simulink model "GFM_29bus"  (R2019a)
settings: Solver=ode1  StartTime=0.0  StopTime=4.5  FixedStep=Time_Step  RelTol=1e-3  EnableMultiTasking=on
PreLoadFcn:
  | Init_29bus;
InitFcn:
  | Init_29bus;
undefined symbols (not defined in the file): D1, D11, Delta, Time_Step, VSC01_Delta_P_Time_Step, VSC01_Delta_P_Value
libraries: powerlib x175, GFM_Lib x1
(part 1 of 5)
Description:
  | Copyright 2008-2017 The MathWorks, Inc.
settings Model: Creator=MathWorks  LastModifiedBy=Frederic_Colas
settings DataIOCC: SaveFormat=StructureWithTime  SignalLoggingSaveFormat=ModelDataLogs  SaveOutput=off  SignalLogging=off  DSMLogging=off  SaveTime=off  ReturnWorkspaceOutputs=off
settings OptimizationCC: ExpressionDepthLimit=2147483647  LifeSpan=inf
settings DebuggingCC: UnderspecifiedInitializationDetection=Classic  MergeDetectMultiDrivingBlocksExec=none  SolverPrmCheckMsg=warning  FcnCallInpInsideContextMsg=warning  UnconnectedInputMsg=none  UnconnectedOutputMsg=none  UnconnectedLineMsg=none  StateNameClashWarn=warning  SFUnexpectedBacktrackingDiag=warning  SFNoUnconditionalDefaultTransitionDiag=warning  SFExecutionAtInitializationDiag=none  ArithmeticOperatorsInVariantConditions=warning
settings HardwareCC: ProdBitPerPointer=32  ProdBitPerSizeT=32  ProdBitPerPtrDiffT=32  ProdLargestAtomicFloat=None  ProdIntDivRoundTo=Undefined  ProdEndianess=Unspecified  ProdWordSize=32  ProdHWDeviceType=32-bit Generic
settings ModelReferenceCC: PropagateSignalLabelsOutOfModel=off
settings SFSimCC: SimUseLocalCustomCode=off
settings RTWCC: RTWUseLocalCustomCode=off
settings CodeAppCC: StateflowObjectComments=on
settings GRTTargetCC: TargetLangStandard=C89/C90 (ANSI)  CombineOutputUpdateFcns=off  GRTInterface=on
settings ConfigComp: CovMetricSettings=dw  CovSaveCumulativeToWorkspaceVar=on  CovSaveSingleToWorkspaceVar=on  CovExternalEMLEnable=off  CovSFcnEnable=off
settings SimscapeCC: SimscapeNormalizeSystem=off

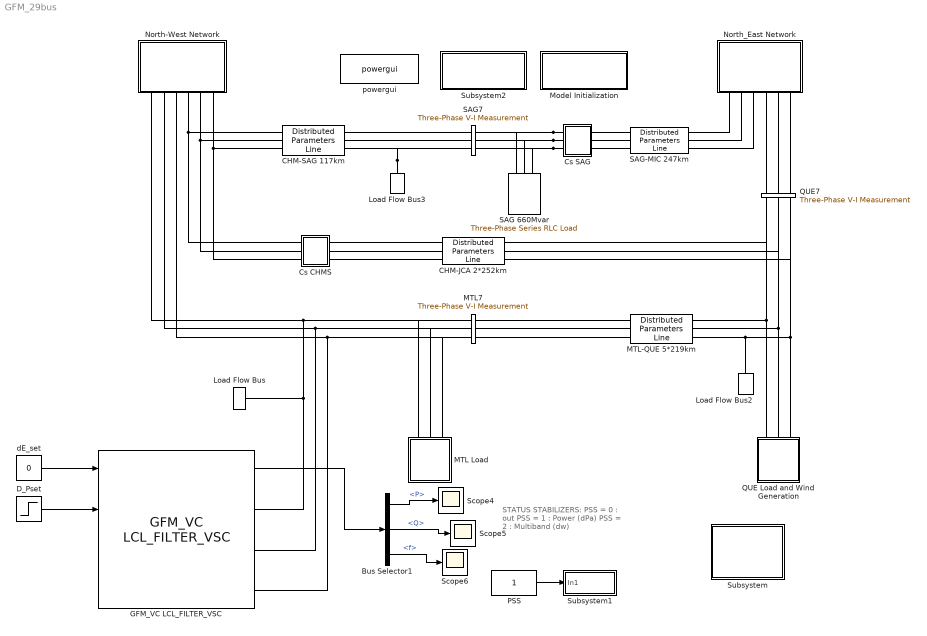
== system GFM_29bus ==
  note: STATUS STABILIZERS:
      | PSS = 0 :  out
      | PSS = 1 :  Power (dPa)
      | PSS = 2 :  Multiband (dw)
  Bus Selector1 : BusSelector  OutputSignals=P,Q,f
  CHM-JCA 2*252km : powerlib/Elements/Distributed Parameters Line  Phases=3  Length=252  Frequency=60  Resistance="[0.01273  0.3864]/2"  Inductance="[0.9337e-3  4.1264e-3]/2"  Capacitance=[12.74e-9 7.751e-9]*2  x1=[-0.00144 -2.67597627648881e-08 0 0;-0.0014 -2.6378453251211e-08 0 0;-0.00136 -2.59911455047426e-08 0 0;-0.00132 -2.55979275959245e-08 0 0;-0.00128 -2.51988889391182e-08 0 0;-0.00124 -2.47941202722731e-08 0 0;-0.0012 -2.43837136362936e-08 0 0;-0.00116 -2.39677623541093e-08 0 0;-0.00112 -2.35463610094548e-08 0 0;-0.00108 -2.3119605425362e-08 0 0;-0.00104 -2.26875926423704e-08 0 0;-0.001 -2.22504208964615e-08 0 0;-0.00096 -2.18081895967201e-08 0 0;-0.00092 -2.13609993027303e-08 0 0;-0.00088 -2.09089517017084e-08 236942.352172574 -735004.326361009;-0.00084 -2.04521495853807e-08 247998.624561456 -731347.868692905;-0.0008 -1.99906968266091e-08 258998.504201761 -727525.108826337;-0.00076 -1.95246983557715e-08 269939.48981572 -723536.916023931;-0.00072 -1.90542601369017e-08 280819.093517553 -719384.197166337;-0.00068 -1.85794891435937e-08 291634.841379201 -715067.896546013;-0.00064 -1.81004933346771e-08 302384.273992871 -710588.995652497;-0.0006 -1.76173816296682e-08 313064.947030286 -705948.512949229;-0.00056 -1.71302638840026e-08 323674.431798503 -701147.503641956;-0.00052 -1.66392508640548e-08 334210.315792179 -696187.059438794;-0.00048 -1.61444542219513e-08 344670.203242151 -691068.308301977;-0.00044 -1.56459864701817e-08 355051.715660215 -685792.414191371;-0.0004 -1.51439609560139e-08 365352.492379973 -680360.576799801;-0.00036 -1.46384918357207e-08 375570.19109363 -674774.031280245;-0.00032 -1.4129694048621e-08 385702.488384611 -669034.04796498;-0.00028 -1.3617683290944e-08 395747.080255891 -663141.932076712;-0.00024 -1.31025759895205e-08 405701.682653897 -657099.023431781;-0.0002 -1.25844892753088e-08 415564.031987891 -650906.696135503;-0.00016 -1.20635409567599e-08 425331.885644682 -644566.358269704;-0.00012 -1.1539849493029e-08 435003.022498583 -638079.451572539;-8e-05 -1.10135339670388e-08 444575.243416475 -631447.451110648;-4e-05 -1.04847140584011e-08 454046.371757867 -624671.864943746]  x2=[-0.00144 -1.4600860870236e-08 0 0;-0.0014 -1.43294294717049e-08 0 0;-0.00136 -1.40547396844836e-08 0 0;-0.00132 -1.37768539706611e-08 0 0;-0.00128 -1.34958355190521e-08 0 0;-0.00124 -1.32117482308293e-08 0 0;-0.0012 -1.2924656704992e-08 0 0;-0.00116 -1.26346262236775e-08 0 0;-0.00112 -1.23417227373161e-08 0 0;-0.00108 -1.20460128496347e-08 0 0;-0.00104 -1.17475638025117e-08 0 0;-0.001 -1.14464434606867e-08 0 0;-0.00096 -1.11427202963286e-08 0 0;-0.00092 -1.08364633734659e-08 0 0;-0.00088 -1.05277423322818e-08 28163.3336001063 -750120.911448412;-0.00084 -1.02166273732786e-08 39471.2795332616 -749610.920406117;-0.0008 -9.90318924131526e-09 50770.2500378369 -748930.474304891;-0.00076 -9.58749920951988e-09 62057.6758253775 -748079.72787231;-0.00072 -9.26962906308333e-09 73330.9902325981 -747058.874560775;-0.00068 -8.94965108293571e-09 84587.6298050193 -745868.146503526;-0.00064 -8.62763802931033e-09 95825.0348798755 -744507.814461855;-0.0006 -8.30366312519867e-09 107040.65016816 -742978.187763538;-0.00056 -7.97780003970008e-09 118231.925335675 -741279.614232494;-0.00052 -7.65012287127008e-09 129396.315582958 -739412.480109697;-0.00048 -7.320706130871e-09 140531.282223944 -737377.209965344;-0.00044 -6.98962472502885e-09 151634.293263242 -735174.266602316;-0.0004 -6.65695393880017e-09 162702.82397189 -732804.150950935;-0.00036 -6.32276941865294e-09 173734.357461457 -730267.401955062;-0.00032 -5.98714715526515e-09 184726.385256358 -727564.596449542;-0.00028 -5.65016346624522e-09 195676.407864264 -724696.349029039;-0.00024 -5.31189497877799e-09 206581.935344464 -721663.311908283;-0.0002 -4.97241861220042e-09 217440.487874052 -718466.174773757;-0.00016 -4.63181156051074e-09 228249.596311826 -715105.664626877;-0.00012 -4.29015127481525e-09 239006.802759738 -711582.545618669;-8e-05 -3.94751544571655e-09 249709.66112181 -707897.618876014;-4e-05 -3.60398198564742e-09 260355.737660347 -704051.722319475]  x3=[-0.00144 -3.6388062339153e-11 0 0;-0.0014 -3.50181673473334e-11 0 0;-0.00136 -3.36403095262429e-11 0 0;-0.00132 -3.22548021888677e-11 0 0;-0.00128 -3.08619603876283e-11 0 0;-0.00124 -2.94621008427391e-11 0 0;-0.0012 -2.80555418701885e-11 0 0;-0.00116 -2.66426033093573e-11 0 0;-0.00112 -2.52236064502896e-11 0 0;-0.00108 -2.37988739606342e-11 0 0;-0.00104 -2.23687298122729e-11 0 0;-0.001 -2.0933499207652e-11 0 0;-0.00096 -1.94935085058341e-11 0 0;-0.00092 -1.80490851482869e-11 0 0;-0.00088 -1.66005575844256e-11 329.791450075946 -923.132329667957;-0.00084 -1.51482551969267e-11 343.673905897847 -918.054417019774;-0.0008 -1.3692508226829e-11 357.478213237264 -912.767746714126;-0.00076 -1.22336476984397e-11 371.201233113752 -907.273520894248;-0.00072 -1.07720053440623e-11 384.839845030933 -901.572988899713;-0.00068 -9.30791352856341e-12 398.390947686072 -895.667446982337;-0.00064 -7.84170517379618e-12 411.851459675284 -889.558238011423;-0.0006 -6.37371368289642e-12 425.218320194221 -883.24675116841;-0.00056 -4.90427286446973e-12 438.488489734073 -876.734421630976;-0.00052 -3.4337168566863e-12 451.658950772723 -870.022730246699;-0.00048 -1.96238005130078e-12 464.726708460909 -863.113203196321;-0.00044 -4.90597017614441e-13 477.688791303222 -856.007411646706;-0.0004 9.81297573602977e-13 490.542251833807 -848.706971393577;-0.00036 2.45296902621451e-12 503.28416728658 -841.213542494091;-0.00032 3.92408269482298e-12 515.91164025985 -833.528828889357;-0.00028 5.3943040608665e-12 528.421799375157 -825.654578016981;-0.00024 6.86329880868507e-12 540.811799930202 -817.592580413706;-0.0002 8.33073290154112e-12 553.078824545706 -809.344669308262;-0.00016 9.79627265757654e-12 565.220083806056 -800.912720204509;-0.00012 1.12595848256891e-11 577.232816893599 -792.298650454959;-8e-05 1.27203366613108e-11 589.114292216425 -783.504418824788;-4e-05 1.41781960020712e-11 600.861808029505 -774.53202504643]  x4=[-0.00144 -9.42654119774044e-11 0 0;-0.0014 -9.45279636497521e-11 0 0;-0.00136 -9.47690204783402e-11 0 0;-0.00132 -9.49885276489247e-11 0 0;-0.00128 -9.51864352474681e-11 0 0;-0.00124 -9.5362698271489e-11 0 0;-0.0012 -9.55172766402959e-11 0 0;-0.00116 -9.56501352041007e-11 0 0;-0.00112 -9.57612437520117e-11 0 0;-0.00108 -9.58505770189034e-11 0 0;-0.00104 -9.5918114691161e-11 0 0;-0.001 -9.59638414113005e-11 0 0;-0.00096 -9.598774678146e-11 0 0;-0.00092 -9.59898253657645e-11 0 0;-0.00088 -9.59700766915618e-11 -191.765553130273 -10272.516028815;-0.00084 -9.59285052495301e-11 -36.8434114817114 -10274.2393304648;-0.0008 -9.58651204926569e-11 118.087108040897 -10273.626358692;-0.00076 -9.57799368340892e-11 272.990775573478 -10270.6772528813;-0.00072 -9.56729736438565e-11 427.832367357865 -10265.3926836338;-0.00068 -9.55442552444657e-11 582.576673751384 -10257.773852615;-0.00064 -9.53938109053709e-11 737.188507233219 -10247.8224922815;-0.0006 -9.52216748363174e-11 891.632710405753 -10235.5408654866;-0.00056 -9.50278861795629e-11 1045.87416398905 -10220.9317649665;-0.00052 -9.48124890009768e-11 1199.8777948067 -10203.9985127045;-0.00048 -9.45755322800199e-11 1353.60858376111 -10184.7449591764;-0.00044 -9.43170698986072e-11 1507.03157379659 -10163.175482474;-0.0004 -9.40371606288553e-11 1660.11187784828 -10139.2949873103;-0.00036 -9.37358681197183e-11 1812.81468677515 -10113.1089039042;-0.00032 -9.34132608825146e-11 1965.10527727529 -10084.623186745;-0.00028 -9.30694122753479e-11 2116.94901978172 -10053.8443132392;-0.00024 -9.27044004864262e-11 2268.31138633685 -10020.7792822373;-0.0002 -9.23183085162826e-11 2419.1579584438 -9985.43561244209;-0.00016 -9.19112241589016e-11 2569.45443489294 -9947.82134069935;-0.00012 -9.14832399817555e-11 2719.16663956161 -9907.9450201701;-8e-05 -9.10344533047553e-11 2868.26052918554 -9865.81571838574;-4e-05 -9.05649661781214e-11 3016.70220109996 -9821.44301518619]  x5=0.00142516474882927  V1=ones(3,3)  V2=ones(3,3)  I1=ones(3,3)  I2=ones(3,3)  nHarmo=1  Measurements=None  Decoupling=off  VsMag0=0  VrMag0=0  VsAngle0=0  VrAngle0=0  IsMag0=0  IrMag0=0  IsAngle0=0  IrAngle0=0
      settings: AttributesFormatString=\n
  CHM-SAG 117km : powerlib/Elements/Distributed Parameters Line  Phases=3  Length=117  Frequency=60  Resistance="[0.01273  0.3864]"  Inductance="[0.9337e-3  4.1264e-3]"  Capacitance=[12.74e-9 7.751e-9]  x1=[-0.00068 -1.88369587854021e-08 0 0;-0.00064 -1.83535071460225e-08 0 0;-0.0006 -1.78658820773917e-08 0 0;-0.00056 -1.73741944612454e-08 0 0;-0.00052 -1.68785561031073e-08 0 0;-0.00048 -1.63790797068658e-08 0 0;-0.00044 -1.58758788491462e-08 285909.998361641 -721015.91713952;-0.0004 -1.53690679534839e-08 296749.772355884 -716622.663851503;-0.00036 -1.48587622643063e-08 307522.068010955 -712066.456749616;-0.00032 -1.43450778207263e-08 318224.435799717 -707348.331876064;-0.00028 -1.38281314301565e-08 328854.44209603 -702469.362091756;-0.00024 -1.33080406417482e-08 339409.669728129 -697430.656832346;-0.0002 -1.27849237196616e-08 349887.718528277 -692233.361855958;-0.00016 -1.22588996161737e-08 360286.205878534 -686878.65898265;-0.00012 -1.17300879446293e-08 370602.767252551 -681367.765825679;-8e-05 -1.11986089522423e-08 380835.056753236 -675701.935514625;-4e-05 -1.06645834927522e-08 390980.747646197 -669882.456410439]  x2=[-0.00068 -1.2548403440967e-08 0 0;-0.00064 -1.22231922766337e-08 0 0;-0.0006 -1.18952016637851e-08 0 0;-0.00056 -1.15645061846579e-08 0 0;-0.00052 -1.12311810365524e-08 0 0;-0.00048 -1.08953020147328e-08 0 0;-0.00044 -1.05569454951921e-08 332770.788350952 -689010.585908437;-0.0004 -1.0216188417285e-08 343122.624715954 -683914.34937034;-0.00036 -9.87310826623243e-09 353396.43795506 -678662.596607021;-0.00032 -9.52778305550223e-09 363589.891891735 -673256.521821772;-0.00028 -9.1802913090693e-09 373700.668622461 -667697.354309377;-0.00024 -8.83071204356015e-09 383726.469043798 -661986.358176588;-0.0002 -8.47912475028511e-09 393665.013375192 -656124.832054678;-0.00016 -8.12560937716272e-09 403514.041677366 -650114.108804138;-0.00012 -7.77024631054023e-09 413271.31436622 -643955.555211601;-8e-05 -7.41311635691447e-09 422934.612722086 -637650.571679046;-4e-05 -7.05430072455714e-09 432501.739394253 -631200.591905354]  x3=[-0.00068 3.06047958909642e-11 0 0;-0.00064 3.14232843209806e-11 0 0;-0.0006 3.22346273671253e-11 0 0;-0.00056 3.30386405369863e-11 0 0;-0.00052 3.38351410049023e-11 0 0;-0.00048 3.46239476535356e-11 0 0;-0.00044 3.54048811150567e-11 1667.27158327278 -3842.29301438702;-0.0004 3.61777638119309e-11 1725.02022392498 -3816.71514574323;-0.00036 3.6942419997298e-11 1782.37660985421 -3790.26938898924;-0.00032 3.76986757949356e-11 1839.32769871292 -3762.96175766209;-0.00028 3.8446359238797e-11 1895.86054031463 -3734.79846128165;-0.00024 3.91853003121147e-11 1951.96227957867 -3705.78590393864;-0.0002 3.99153309860611e-11 2007.62015945335 -3675.93068283841;-0.00016 4.06362852579565e-11 2062.82152381674 -3645.23958680079;-0.00012 4.13479991890166e-11 2117.55382035463 -3613.71959471633;-8e-05 4.2050310941631e-11 2171.80460341478 -3581.37787395942;-4e-05 4.27430608161638e-11 2225.56153683696 -3548.22177875846]  x4=[-0.00068 -8.16423559054635e-11 0 0;-0.00064 -8.15296698683215e-11 0 0;-0.0006 -8.13984446873333e-11 0 0;-0.00056 -8.12487102019735e-11 0 0;-0.00052 -8.10805004605728e-11 0 0;-0.00048 -8.08938537125758e-11 0 0;-0.00044 -8.06888123998435e-11 212.776929450968 -1518.35868415078;-0.0004 -8.04654231470021e-11 235.648399149778 -1514.97750591382;-0.00036 -8.02237367508413e-11 258.466284434767 -1511.25183485662;-0.00032 -7.99638081687635e-11 281.225396715594 -1507.18251816465;-0.00028 -7.96856965062865e-11 303.920560766392 -1502.77048116544;-0.00024 -7.93894650036043e-11 326.546615902571 -1498.01672711816;-0.0002 -7.90751810212058e-11 349.098417154312 -1492.92233698547;-0.00016 -7.87429160245584e-11 371.570836436488 -1487.48846918777;-0.00012 -7.8392745567857e-11 393.95876371475 -1481.71635933972;-8e-05 -7.80247492768437e-11 416.257108167498 -1475.60731996935;-4e-05 -7.76390108307016e-11 438.460799343497 -1469.1627402195]  x5=0.000661683633385019  V1=ones(3,3)  V2=ones(3,3)  I1=ones(3,3)  I2=ones(3,3)  nHarmo=1  Measurements=None  Decoupling=off  VsMag0=0  VrMag0=0  VsAngle0=0  VrAngle0=0  IsMag0=0  IrMag0=0  IsAngle0=0  IrAngle0=0
      settings: AttributesFormatString=\n
  Cs CHMS : Subsystem  mask{Xc=33/2}
      mask prompts: Xc "Condensator Reactance at  60Hz  (ohm):"
      mask help: Series Compensation
      mask init:
      | Cs=1/Xc/(2*pi*60);
      mask Display: disp('Cs')
  Cs SAG : Subsystem  mask{Xc=22}
      mask prompts: Xc "Condensator Reactance at  60Hz  (ohm):"
      mask help: Series Compensation
      mask init:
      | Cs=1/Xc/(2*pi*60);
      mask Display: disp('Cs')
  D_Pset : Step  Time=VSC01_Delta_P_Time_Step  After=VSC01_Delta_P_Value  SampleTime=0
  GFM_VC LCL_FILTER_VSC : GFM_Lib/GFM_VC LCL_FILTER_VSC  fn=fb  Sn=VSC01_Sn  Pn=VSC01_Pn  Udcn=VSC01_Udc_n  bridge_type=Average (no switches)  Output_Delay=0.0001  fpwm=5000  Tcontroller=50e-6  Un1=VSC01_Un1  Un2=VSC01_Un2  Rt_pu=VSC01_Rt_pu  Lt_pu=VSC01_Lt_pu  Rm_pu=500  Lm_pu=500  Lf_pu=VSC01_Lf_pu  Rf_pu=VSC01_Rf_pu  Cf_pu=VSC01_Cf_pu  DC_Link=Perfect DC Source  H_DC=inf  H_DC_sav=inf  wn_PLL=50  zeta_PLL=1  Val_Freq_Support=on  Val_gamma=on  R_percent=4  dLc_pu=0  Rv=0.09  W_TVR=60  RLCL_D=0.7  f_damping=200  I_max_pu=1.2  wn_I_max=300  I_Max_TVI_pu=1.2  DX_DR=5  Advanced=off  gainpopup=With Inertia  wn_Inertia_Less=3  Param_Inertia=PI  H_GFo=5  zeta_GFo=1  LFpopup=PV  P0=0.9  Q0=-0.3128  V0=1  Theta0=-17.0119
      settings: SourceProductName=VSC4SPS
  Load Flow Bus : powerlib/Measurements/Load Flow Bus  LConnTagsString=a  Phases=single  Connectors=on one side  ID=BUS_1  Vbase=VSC01_Un2  Vref=1  Vangle=0  VLF=1  VLFb=1  VLFc=1  angleLF=-17.01  angleLFb=0  angleLFc=0
  Load Flow Bus2 : powerlib/Measurements/Load Flow Bus  LConnTagsString=a  Phases=single  Connectors=on one side  ID=QUE7  Vbase=735e3  Vref=1  Vangle=0  VLF=1.021  VLFb=1  VLFc=1  angleLF=-8.842  angleLFb=0  angleLFc=0
      settings: AttributesFormatString=%<ID>\n%<Vbase>V\n%<VLF>pu\n%<angleLF>deg.
  Load Flow Bus3 : powerlib/Measurements/Load Flow Bus  LConnTagsString=a  Phases=single  Connectors=on one side  ID=SAG7  Vbase=735e3  Vref=1  Vangle=0  VLF=1.041  VLFb=1  VLFc=1  angleLF=5.283  angleLFb=0  angleLFc=0
      settings: AttributesFormatString=%<ID>\n%<Vbase>V\n%<VLF>pu\n%<angleLF>deg.
  MTL Load : Subsystem
  MTL-QUE 5*219km : powerlib/Elements/Distributed Parameters Line  Phases=3  Length=219  Frequency=60  Resistance="[0.01273  0.3864]/5"  Inductance="[0.9337e-3  4.1264e-3]/5"  Capacitance=[12.74e-9 7.751e-9]*5  x1=[-0.00124 -9.89581855731986e-08 -175266.105408257 -713798.743426965;-0.0012 -9.73562168099365e-08 -164482.743702122 -716360.413325681;-0.00116 -9.5732110082536e-08 -153661.980038508 -718759.189044035;-0.00112 -9.40862346988612e-08 -142806.274965757 -720994.525121116;-0.00108 -9.24189649167812e-08 -131918.096977589 -723065.913260777;-0.00104 -9.07306798590662e-08 -120999.921951781 -724972.882447216;-0.001 -8.90217634271793e-08 -110054.23258718 -726714.999052087;-0.00096 -8.72926042139801e-08 -99083.5178391556 -728291.866933097;-0.00092 -8.5543595415362e-08 -88090.2723536348 -729703.127524088;-0.00088 -8.3775134740843e-08 -77076.9958998388 -730948.459916572;-0.00084 -8.19876243231299e-08 -66046.192801859 -732027.580932702;-0.0008 -8.01814706266769e-08 -55000.3713691941 -732940.245189664;-0.00076 -7.8357084355259e-08 -43942.0433263829 -733686.245155478;-0.00072 -7.65148803585813e-08 -32873.7232418593 -734265.411196185;-0.00068 -7.46552775379464e-08 -21797.9279561614 -734677.61161442;-0.00064 -7.2778698750999e-08 -10717.1760096237 -734922.752679364;-0.0006 -7.08855707155724e-08 366.012930317724 -735000.778648053;-0.00056 -6.89763239126562e-08 11449.1186420751 -734911.671778054;-0.00052 -6.70513924885088e-08 22529.6209229862 -734655.452331502;-0.00048 -6.5111214155936e-08 33605.0001623868 -734232.178570487;-0.00044 -6.31562300947594e-08 44672.7379145475 -733641.946743815;-0.0004 -6.11868848514954e-08 55730.3174713477 -732884.891065111;-0.00036 -5.92036262382694e-08 66775.2244345527 -731961.18368231;-0.00032 -5.72069052309871e-08 77804.9472875664 -730871.034638503;-0.00028 -5.51971758667866e-08 88816.9779665281 -729614.691824183;-0.00024 -5.31748951407942e-08 99808.8124306252 -728192.440920872;-0.0002 -5.11405229022076e-08 110777.95123149 -726604.605336159;-0.00016 -4.909452174973e-08 121721.900081553 -724851.546130164;-0.00012 -4.70373569263797e-08 132638.170421223 -722933.661933432;-8e-05 -4.49694962136973e-08 143524.279984762 -720851.388856292;-4e-05 -4.28914098253762e-08 154377.753364733 -718605.200389683]  x2=[-0.00124 -1.32117482308293e-08 -73587.5945080477 -747034.022065887;-0.0012 -1.2924656704992e-08 -62314.6314105149 -748058.689266913;-0.00116 -1.26346262236775e-08 -51027.4985031779 -748913.254372983;-0.00112 -1.23417227373161e-08 -39728.7623827236 -749597.523063362;-0.00108 -1.20460128496347e-08 -28420.9922843098 -750111.33974125;-0.00104 -1.17475638025117e-08 -17106.7594973426 -750454.587569166;-0.001 -1.14464434606867e-08 -5788.63678078831 -750627.188495513;-0.00096 -1.11427202963286e-08 5530.80222185096 -750629.103272329;-0.00092 -1.08364633734659e-08 16848.9835677605 -750460.331464211;-0.00088 -1.05277423322818e-08 28163.3336001063 -750120.911448412;-0.00084 -1.02166273732786e-08 39471.2795332616 -749610.920406117;-0.0008 -9.90318924131526e-09 50770.2500378369 -748930.474304891;-0.00076 -9.58749920951988e-09 62057.6758253775 -748079.72787231;-0.00072 -9.26962906308333e-09 73330.9902325981 -747058.874560775;-0.00068 -8.94965108293571e-09 84587.6298050193 -745868.146503526;-0.00064 -8.62763802931033e-09 95825.0348798755 -744507.814461855;-0.0006 -8.30366312519867e-09 107040.65016816 -742978.187763538;-0.00056 -7.97780003970008e-09 118231.925335675 -741279.614232494;-0.00052 -7.65012287127008e-09 129396.315582958 -739412.480109697;-0.00048 -7.320706130871e-09 140531.282223944 -737377.209965344;-0.00044 -6.98962472502885e-09 151634.293263242 -735174.266602316;-0.0004 -6.65695393880017e-09 162702.82397189 -732804.150950935;-0.00036 -6.32276941865294e-09 173734.357461457 -730267.401955062;-0.00032 -5.98714715526515e-09 184726.385256358 -727564.596449542;-0.00028 -5.65016346624522e-09 195676.407864264 -724696.349029039;-0.00024 -5.31189497877799e-09 206581.935344464 -721663.311908283;-0.0002 -4.97241861220042e-09 217440.487874052 -718466.174773757;-0.00016 -4.63181156051074e-09 228249.596311826 -715105.664626877;-0.00012 -4.29015127481525e-09 239006.802759738 -711582.545618669;-8e-05 -3.94751544571655e-09 249709.66112181 -707897.618876014;-4e-05 -3.60398198564742e-09 260355.737660347 -704051.722319475]  x3=[-0.00124 6.71653303483164e-10 -7027.02739090939 -19339.02688402;-0.0012 6.92523500703499e-10 -6734.61410510097 -19442.7883835754;-0.00116 7.13236224051843e-10 -6440.66942612189 -19542.1287607198;-0.00112 7.33786763633524e-10 -6145.26019445728 -19637.0254263082;-0.00108 7.54170446433062e-10 -5848.45358361892 -19727.4568016571;-0.00104 7.74382637376771e-10 -5550.31708487055 -19813.4023234516;-0.001 7.94418740386732e-10 -5250.91849188099 -19894.8424484214;-0.00096 8.14274199425904e-10 -4950.32588530836 -19971.7586577841;-0.00092 8.33944499534128e-10 -4648.60761731921 -20044.1334614572;-0.00088 8.53425167854789e-10 -4345.83229604576 -20111.9504020344;-0.00084 8.72711774651905e-10 -4042.06876998505 -20175.1940585282;-0.0008 8.91799934317412e-10 -3737.38611234336 -20233.8500498766;-0.00076 9.10685306368409e-10 -3431.85360532958 -20287.905038213;-0.00072 9.29363596434154e-10 -3125.54072440098 -20337.3467318991;-0.00068 9.4783055723256e-10 -2818.51712246517 -20382.1638883202;-0.00064 9.66081989535994e-10 -2510.85261404157 -20422.3463164413;-0.0006 9.84113743126144e-10 -2202.61715938621 -20457.884879125;-0.00056 1.00192171773774e-09 -1893.88084858337 -20488.7714952084;-0.00052 1.01950186399093e-09 -1584.71388560769 -20514.9991413414;-0.00048 1.03685018431206e-09 -1275.18657236041 -20536.5618535835;-0.00044 1.05396273384269e-09 -965.369292683318 -20553.4547287599;-0.0004 1.07083562133663e-09 -655.332496354061 -20565.6739255764;-0.00036 1.08746501004478e-09 -345.14668306648 -20573.216665493;-0.00032 1.10384711858753e-09 -34.8823863995876 -20576.0812333558;-0.00028 1.1199782218147e-09 275.389842221159 -20574.2669777866;-0.00024 1.1358546516525e-09 585.599449566646 -20567.7743113317;-0.0002 1.15147279793771e-09 895.675896647295 -20556.6047103672;-0.00016 1.16682910923855e-09 1205.54867475303 -20540.7607147643;-0.00012 1.18192009366225e-09 1515.14732148633 -20520.2459273108;-8e-05 1.1967423196491e-09 1824.4014367848 -20495.0650128924;-4e-05 1.21129241675273e-09 2133.24069892951 -20465.2236974321]  x4=[-0.00124 -1.55492946416296e-09 -1381.21463376686 -6777.21285106667;-0.0012 -1.56656659207367e-09 -1278.86289977349 -6797.26945353827;-0.00116 -1.57784749625084e-09 -1176.22036338515 -6815.78041555329;-0.00112 -1.58876961151413e-09 -1073.31036462947 -6832.74152787859;-0.00108 -1.59933045426874e-09 -970.156304352711 -6848.14893370351;-0.00104 -1.60952762307008e-09 -866.781638898612 -6861.99912951683;-0.001 -1.61935879916991e-09 -763.209874774634 -6874.28896590346;-0.00096 -1.62882174704356e-09 -659.464563306774 -6885.01564826058;-0.00092 -1.6379143148983e-09 -555.569295284198 -6894.17673743314;-0.00088 -1.6466344351626e-09 -451.547695594899 -6901.77015026844;-0.00084 -1.65498012495631e-09 -347.423417853604 -6907.79416008991;-0.0008 -1.66294948654156e-09 -243.220139023142 -6912.24739708966;-0.00076 -1.67054070775422e-09 -138.961554030506 -6915.12884863999;-0.00072 -1.67775206241608e-09 -34.6713703788371 -6916.43785952367;-0.00068 -1.68458191072725e-09 69.6266972434626 -6916.17413208292;-0.00064 -1.69102869963915e-09 173.908932355244 -6914.33772628707;-0.0006 -1.69709096320755e-09 278.151622075535 -6910.92905971898;-0.00056 -1.70276732292601e-09 382.331062515643 -6905.94890748002;-0.00052 -1.70805648803928e-09 486.423564169218 -6899.39840201386;-0.00048 -1.71295725583682e-09 590.405457299039 -6891.27903284897;-0.00044 -1.7174685119263e-09 694.25309731931 -6881.59264625986;-0.0004 -1.72158923048698e-09 797.942870172235 -6870.34144484733;-0.00036 -1.72531847450301e-09 901.451197697648 -6857.52798703753;-0.00032 -1.72865539597644e-09 1004.75454299449 -6843.15518650029;-0.00028 -1.73159923612012e-09 1107.82941577289 -6827.22631148649;-0.00024 -1.73414932553018e-09 1210.65237769565 -6809.74498408495;-0.0002 -1.73630508433828e-09 1313.20004770795 -6790.71517939878;-0.00016 -1.73806602234346e-09 1415.44910735396 -6770.14122464144;-0.00012 -1.7394317391236e-09 1517.37630607926 -6748.02779815283;-8e-05 -1.74040192412649e-09 1618.95846651786 -6724.37992833543;-4e-05 -1.74097635674042e-09 1720.17248976248 -6699.20299251091]  x5=0.00123853603172068  V1=ones(3,3)  V2=ones(3,3)  I1=ones(3,3)  I2=ones(3,3)  nHarmo=1  Measurements=None  Decoupling=off  VsMag0=0  VrMag0=0  VsAngle0=0  VrAngle0=0  IsMag0=0  IrMag0=0  IsAngle0=0  IrAngle0=0
      settings: AttributesFormatString=\n
  MTL7 : powerlib/Measurements/Three-Phase V-I Measurement  VoltageMeasurement=phase-to-ground  SetLabelV=on  LabelV=Vabc_MTL7  Vpu=on  VpuLL=off  CurrentMeasurement=no  SetLabelI=off  LabelI=A1  Ipu=off  Pbase=100e6  Vbase=735e3  OutputType=Magnitude  PhasorSimulation=off  PSBequivalent=0
  Model Initialization : Subsystem  mask(Model Functions){InitFcnX=Init_29bus;, prel=on, posl=off, inif=on, strf=off}
      mask prompts: InitFcnX "Initialisation"; prel "Preload Function"; posl "PostLoad Function"; inif "InitFcn"; strf "StartFcn"
      mask init:
      | currentBlock = gcb;
      | root = bdroot(currentBlock);
      | 
      | if ~strcmp(get_param(root,'BlockDiagramType'),'library')
      |     if prel==1
      |         set_param(root, 'PreLoadFcn', InitFcnX);
      |     else
      |         set_param(root, 'PreLoadFcn', '');
      |     end
      |     if inif==1
      |         set_param(root, 'InitFcn', InitFcnX);
      |     else
      |         set_param(root, 'InitFcn', '');
      |     end
      |     if strf==1
      |         set_param(root, 'StartFcn', InitFcnX);
      |     else
      |         set_param(root, 'StartFcn', '');
      |     end
      |     if posl==1
      |         set_param(root, 'PostLoadFcn', InitFcnX);
      |     else
      |         set_param(root, 'PostLoadFcn', '');
      |     end
      | end
      | 
      | pos = get_param(currentBlock, 'Position');
      | width = pos(3) - pos(1); height = pos(4) - pos(2);
      | txt = [ upper(root) '\n' '- InitFcn. . . . . '  get_param(root, 'InitFcn') ];
      settings: CopyFcn=set_param(gcb,'LinkStatus','none')
      mask Display:
      | %text(5, height*0.5, txt, 'horizontalAlignment', 'left', 'verticalAlignment', 'middle') ;
      | color('blue'),disp('Initialization Function\nParameters')
  North-West Network : Subsystem
  North_East Network : Subsystem
  PSS : Constant
  QUE Load and Wind Generation : Subsystem
  QUE7 : powerlib/Measurements/Three-Phase V-I Measurement  VoltageMeasurement=no  SetLabelV=on  LabelV=Vabc_QUE7  Vpu=on  VpuLL=off  CurrentMeasurement=no  SetLabelI=off  LabelI=A1  Ipu=off  Pbase=100e6  Vbase=735e3  OutputType=Magnitude  PhasorSimulation=off  PSBequivalent=0
  SAG 660Mvar : powerlib/Elements/Three-Phase Series RLC Load  LConnTagsString=A|B|C  Configuration=Y (grounded)  NominalVoltage=735e3  Vabc=[1e3 1e3 1e3]  Vabcp=[1e3 1e3 1e3]  NominalFrequency=60  UnbalancedPower=off  ActivePower=2200000  InductivePower=660e6  CapacitivePower=0  Pabc=[10e3 9e3 11e3]  QLabc=[100 90 110]  QCabc=[100 90 110]  Pabcp=[10e3 9e3 11e3]  QLabcp=[100 90 110]  QCabcp=[100 90 110]  Measurements=None  LoadType=constant Z
  SAG-MIC 247km : powerlib/Elements/Distributed Parameters Line  Phases=3  Length=247  Frequency=60  Resistance="[0.01273  0.3864]/1"  Inductance="[0.9337e-3  4.1264e-3]/1"  Capacitance=[12.74e-9 7.751e-9]*1  x1=[-0.0014 -1.86983980919344e-08 36517.9763333113 -754648.034723366;-0.00136 -1.84217395435702e-08 47893.2367885114 -754011.547608988;-0.00132 -1.8140892050496e-08 59257.6067346796 -753203.604771002;-0.00128 -1.78559194750099e-08 70608.5020120922 -752224.389928643;-0.00124 -1.75668866174181e-08 81943.3415250489 -751074.12574692;-0.0012 -1.72738592012999e-08 93259.5478287922 -749753.073785991;-0.00116 -1.69769038585628e-08 104554.547715595 -748261.534441677;-0.00112 -1.66760881142907e-08 115825.772799888 -746599.846877164;-0.00108 -1.637148037139e-08 127070.660102285 -744768.388945874;-0.00104 -1.60631498950344e-08 138286.652632385 -742767.577105547;-0.001 -1.57511667969154e-08 149471.19997021 -740597.86632354;-0.00096 -1.54356020192991e-08 160621.758846146 -738259.749973376;-0.00092 -1.51165273188945e-08 171735.793719264 -735753.759722549;-0.00088 -1.4794015250537e-08 182810.777353877 -733080.465411631;-0.00084 -1.44681391506897e-08 193844.191394212 -730240.474924695;-0.0008 -1.41389731207674e-08 204833.526937065 -727234.434051087;-0.00076 -1.38065920102868e-08 215776.285102302 -724063.026338578;-0.00072 -1.3471071399846e-08 226669.977601082 -720726.972937934;-0.00068 -1.31324875839385e-08 237512.127301675 -717227.032438928;-0.00064 -1.27909175536041e-08 248300.268792736 -713564.000697848;-0.0006 -1.24464389789222e-08 259031.948943924 -709738.710656523;-0.00056 -1.209913019135e-08 269704.727463718 -705752.032152921;-0.00052 -1.17490701659108e-08 280316.177454322 -701604.871723354;-0.00048 -1.13963385032355e-08 290863.885963517 -697298.172396339;-0.00044 -1.10410154114624e-08 301345.454533347 -692832.913478165;-0.0004 -1.06831816879984e-08 311758.499745508 -688210.110330203;-0.00036 -1.03229187011464e-08 322100.653763318 -683430.814138022;-0.00032 -9.96030837160278e-09 332369.56487014 -678496.111672363;-0.00028 -9.59543315382952e-09 342562.898004144 -673407.125042011;-0.00024 -9.22837601730458e-09 352678.335289278 -668165.01143864;-0.0002 -8.85922042765542e-09 362713.576562335 -662770.962873678;-0.00016 -8.48805032767967e-09 372666.339895991 -657226.205907251;-0.00012 -8.11495011825725e-09 382534.362117693 -651532.001369279;-8e-05 -7.74000463915827e-09 392315.399324285 -645689.644072768;-4e-05 -7.36329914975131e-09 402007.227392254 -639700.462519385]  x2=[-0.0014 -7.37879736468657e-09 154416.562837981 -749556.909357134;-0.00136 -7.28991746834684e-09 165701.648163813 -747143.188379854;-0.00132 -7.19937990764038e-09 176949.054363803 -744559.573484626;-0.00128 -7.10720527002772e-09 188156.223874775 -741806.652163195;-0.00124 -7.0134145152266e-09 199320.608283027 -738885.05040613;-0.0012 -6.91802897044581e-09 210439.668903824 -735795.432560477;-0.00116 -6.8210703255357e-09 221510.877358667 -732538.501178689;-0.00112 -6.72256062805595e-09 232531.716150226 -729114.996858875;-0.00108 -6.62252227826229e-09 243499.679234801 -725525.698076396;-0.00104 -6.52097802401274e-09 254412.27259217 -721771.421006842;-0.001 -6.41795095559506e-09 265267.014792709 -717853.019340442;-0.00096 -6.31346450047612e-09 276061.43756165 -713771.384087945;-0.00092 -6.20754241797478e-09 286793.086340342 -709527.443378008;-0.00088 -6.10020879385915e-09 297459.520844398 -705122.162246152;-0.00084 -5.99148803486976e-09 308058.315618596 -700556.542415315;-0.0008 -5.88140486316963e-09 318587.060588404 -695831.622068076;-0.00076 -5.76998431072269e-09 329043.361608012 -690948.475610574;-0.00072 -5.65725171360173e-09 339424.841004739 -685908.213428204;-0.00068 -5.54323270622714e-09 349729.138119697 -680711.981633122;-0.00064 -5.42795321553797e-09 359953.909844582 -675360.961803626;-0.0006 -5.31143945509626e-09 370096.831154479 -669856.370715481;-0.00056 -5.19371791912636e-09 380155.595636551 -664199.46006523;-0.00052 -5.07481537649036e-09 390127.916014497 -658391.516185573;-0.00048 -4.9547588646011e-09 400011.524668661 -652433.859752862;-0.00044 -4.83357568327405e-09 409804.174151668 -646327.845486793;-0.0004 -4.7112933885196e-09 419503.637699474 -640074.861842354;-0.00036 -4.58793978627707e-09 429107.709737712 -633676.330694103;-0.00032 -4.46354292609185e-09 438614.206383223 -627133.707012844;-0.00028 -4.33813109473718e-09 448020.96594065 -620448.478534781;-0.00024 -4.21173280978203e-09 457325.849393991 -613622.165423219;-0.0002 -4.08437681310636e-09 466526.740892989 -606656.319922892;-0.00016 -3.95609206436556e-09 475621.548234264 -599552.526006996;-0.00012 -3.82690773440521e-09 484608.203337056 -592312.399017007;-8e-05 -3.6968531986279e-09 493484.662713492 -584937.585295365;-4e-05 -3.56595803031353e-09 502248.907933257 -577429.761811114]  x3=[-0.0014 6.44908978866869e-12 -207.556751541969 -4152.72851108877;-0.00136 6.99572718557546e-12 -144.913933998385 -4155.38601545119;-0.00132 7.54077381444881e-12 -82.238164275894 -4157.09862086822;-0.00128 8.08410573638563e-12 -19.5436943040379 -4157.86593790816;-0.00124 8.62559940239234e-12 43.1552197353644 -4157.68779208972;-0.0012 9.16513168147896e-12 105.844320649955 -4156.56422392174;-0.00116 9.70257988865793e-12 168.509353478791 -4154.49548889392;-0.00112 1.02378218128417e-11 231.136068733809 -4151.48205741877;-0.00108 1.07707357446325e-11 293.71022564003 -4147.52461472462;-0.00104 1.13012005039978e-11 356.217595373789 -4142.62406069981;-0.001 1.18290954678258e-11 418.64396429825 -4136.78150968806;-0.00096 1.23543005973543e-11 480.975137195461 -4129.9982902351;-0.00092 1.28766964654659e-11 543.196940494227 -4122.27594478652;-0.00088 1.33961642838452e-11 605.295225493056 -4113.6162293371;-0.00084 1.39125859299898e-11 667.255871577451 -4104.02111303144;-0.0008 1.44258439740711e-11 729.064789430819 -4093.49277771624;-0.00076 1.49358217056358e-11 790.707924238257 -4082.03361744418;-0.00072 1.54424031601457e-11 852.171258882499 -4069.64623792946;-0.00068 1.59454731453466e-11 913.440817131282 -4056.33345595537;-0.00064 1.64449172674622e-11 974.502666815428 -4042.09829873373;-0.0006 1.6940621957206e-11 1035.34292299689 -4026.94400321653;-0.00056 1.74324744956065e-11 1095.94775112609 -4010.87401535988;-0.00052 1.7920363039638e-11 1156.30337018772 -3993.89198934044;-0.00048 1.84041766476528e-11 1216.39605583452 -3976.00178672449;-0.00044 1.88838053046089e-11 1276.21214350796 -3957.20747558981;-0.0004 1.93591399470857e-11 1335.73803154556 -3937.51332960069;-0.00036 1.98300724880846e-11 1394.9601842737 -3916.92382703608;-0.00032 2.0296495841607e-11 1453.86513508557 -3895.44364977132;-0.00028 2.07583039470045e-11 1512.43948950331 -3873.07768221348;-0.00024 2.12153917930965e-11 1570.66992822386 -3849.8310101907;-0.0002 2.16676554420485e-11 1628.54321014761 -3825.70891979573;-0.00016 2.21149920530069e-11 1686.04617538933 -3800.71689618391;-0.00012 2.25572999054839e-11 1743.16574827062 -3774.86062232589;-8e-05 2.29944784224884e-11 1799.88894029317 -3748.14597771536;-4e-05 2.34264281933955e-11 1856.20285309227 -3720.57903703213]  x4=[-0.0014 -4.77777152706726e-11 11.9116888500906 -1468.5914323996;-0.00136 -4.80119768925544e-11 34.0555064809955 -1468.24467358199;-0.00132 -4.82353210049285e-11 56.1915801834091 -1467.5640485872;-0.00128 -4.84476968212698e-11 78.3148764050645 -1466.5497121835;-0.00124 -4.86490560491491e-11 100.420364499184 -1465.20189502224;-0.0012 -4.88393529012144e-11 122.503017868405 -1463.52090358541;-0.00116 -4.90185441056025e-11 144.557815107783 -1461.50712011597;-0.00112 -4.9186588915779e-11 166.57974114662 -1459.16100253092;-0.00108 -4.93434491198032e-11 188.563788388842 -1456.48308431716;-0.00104 -4.94890890490172e-11 210.504957851689 -1453.4739744102;-0.001 -4.96234755861573e-11 232.398260302439 -1450.13435705569;-0.00096 -4.97465781728837e-11 254.238717392913 -1446.46499165381;-0.00092 -4.98583688167298e-11 276.021362791513 -1442.46671258661;-0.00088 -4.99588220974672e-11 297.741243312521 -1438.14042902827;-0.00084 -5.00479151728862e-11 319.393420042411 -1433.48712473837;-0.0008 -5.01256277839897e-11 340.972969462915 -1428.50785783816;-0.00076 -5.01919422596002e-11 362.474984570589 -1423.20376057001;-0.00072 -5.02468435203776e-11 383.894575992622 -1417.5760390399;-0.00068 -5.02903190822489e-11 405.226873098641 -1411.62597294316;-0.00064 -5.03223590592461e-11 426.467025108245 -1405.35491527352;-0.0006 -5.03429561657548e-11 447.610202194034 -1398.7642920154;-0.00056 -5.03521057181706e-11 468.65159657987 -1391.85560181972;-0.00052 -5.03498056359641e-11 489.586423634123 -1384.63041566303;-0.00048 -5.03360564421542e-11 510.409922957655 -1377.09037649036;-0.00044 -5.0310861263189e-11 531.117359466295 -1369.23719884161;-0.0004 -5.0274225828235e-11 551.704024467552 -1361.07266846163;-0.00036 -5.02261584678741e-11 572.165236731339 -1352.59864189424;-0.00032 -5.01666701122096e-11 592.496343554436 -1343.81704605999;-0.00028 -5.00957742883804e-11 612.692721818479 -1334.72987781806;-0.00024 -5.00134871174857e-11 632.749779041218 -1325.33920351212;-0.0002 -4.99198273109183e-11 652.662954420805 -1315.64715850055;-0.00016 -4.98148161661108e-11 672.427719872882 -1305.6559466708;-0.00012 -4.96984775616917e-11 692.039581060229 -1295.36783993827;-8e-05 -4.95708379520565e-11 711.494078414739 -1284.78517772971;-4e-05 -4.94319263613517e-11 730.786788151481 -1273.91036645125]  x5=0.00139688767047948  V1=ones(3,3)  V2=ones(3,3)  I1=ones(3,3)  I2=ones(3,3)  nHarmo=1  Measurements=None  Decoupling=off  VsMag0=0  VrMag0=0  VsAngle0=0  VrAngle0=0  IsMag0=0  IrMag0=0  IsAngle0=0  IrAngle0=0
      settings: AttributesFormatString=\n
  SAG7 : powerlib/Measurements/Three-Phase V-I Measurement  VoltageMeasurement=no  SetLabelV=on  LabelV=Vabc_SAG7  Vpu=on  VpuLL=off  CurrentMeasurement=no  SetLabelI=off  LabelI=Iabc_SAG7  Ipu=off  Pbase=100e6  Vbase=735e3  OutputType=Magnitude  PhasorSimulation=off  PSBequivalent=0
  Scope4 : Scope
  Scope5 : Scope
  Scope6 : Scope
  Subsystem : Subsystem
      mask Display: disp('Display\nWaveforms')
  Subsystem1 : Subsystem
      mask Display: disp('PSS_select')
  Subsystem2 : Subsystem
      settings: OpenFcn=LoadFlow_VSC
      mask Display: color('blue'),disp('Update Loadflow')
  dE_set : Constant  Value=0
  powergui : powerlib/powergui  Priority=1  SimulationMode=Discrete  SampleTime=Time_Step  frequency=60  Iterations=50  frequencyindice=60  Pbase=5500000000  ErrMax=1e-6  UnitsV=kV  UnitsW=MW  buscounter=0  FunctionMessages=off  echomessages=off  EnableUseOfTLC=off  CurrentSourceSwitches=off  DisableSnubberDevices=off  DisableRonSwitches=off  DisableVfSwitches=off  DisplayEquations=off  AutomaticDiscreteSolvers=off  SolverType=Tustin/Backward Euler (TBE)  Interpol=off  ExternalGateDelay=off  methode=off  Ts=100  x0status=blocks  SPID=off  SwTol=0  HookPort=off  NonlinearTolerance=1e-4  nMaxIteration=100  ContinueOnMaxIteration=off  RestoreLinks=warning  ResistiveCurrentMeasurement=off  Frange=[0:2:500]  Ylog=off  Xlog=on  ShowGrid=off  save=off  variable=ZData  structure=0  ZoomFFT=off  StartTime=0.0  cycles=1  DisplayStyle=1  fundamental=60  FreqAxis=off  MaxFrequency=1000  frequencyindicesteady=1  RmsSteady=1  display=off
  wires:
  PSS/1 -> Subsystem1/1(In1)
  D_Pset/1 -> GFM_VC LCL_FILTER_VSC/2
  dE_set/1 -> GFM_VC LCL_FILTER_VSC/1
  Bus Selector1/3 -> Scope6/1  "<f>"
  Bus Selector1/2 -> Scope5/1  "<Q>"
  GFM_VC LCL_FILTER_VSC/1 -> Bus Selector1/1
  Bus Selector1/1 -> Scope4/1  "<P>"
  connections:
  QUE Load and Wind Generation/LConn3 -- MTL-QUE 5*219km/RConn3 -- Load Flow Bus2/LConn1 -- CHM-JCA 2*252km/RConn3 -- QUE7/LConn3
  MTL7/RConn1 -- MTL-QUE 5*219km/LConn1
  MTL7/RConn2 -- MTL-QUE 5*219km/LConn2
  MTL7/RConn3 -- MTL-QUE 5*219km/LConn3
  QUE Load and Wind Generation/LConn2 -- MTL-QUE 5*219km/RConn2 -- CHM-JCA 2*252km/RConn2 -- QUE7/LConn2
  QUE Load and Wind Generation/LConn1 -- MTL-QUE 5*219km/RConn1 -- CHM-JCA 2*252km/RConn1 -- QUE7/LConn1
  Cs SAG/LConn1 -- SAG7/RConn1 -- SAG 660Mvar/LConn1
  Cs SAG/LConn2 -- SAG7/RConn2 -- SAG 660Mvar/LConn2
  Cs SAG/LConn3 -- SAG7/RConn3 -- SAG 660Mvar/LConn3
  Load Flow Bus3/LConn1 -- CHM-SAG 117km/RConn3 -- SAG7/LConn3
  Cs CHMS/LConn1 -- CHM-SAG 117km/LConn1 -- North-West Network/RConn4
  Cs CHMS/LConn2 -- CHM-SAG 117km/LConn2 -- North-West Network/RConn5
  Cs CHMS/LConn3 -- CHM-SAG 117km/LConn3 -- North-West Network/RConn6
  Cs SAG/RConn1 -- SAG-MIC 247km/LConn1
  Cs SAG/RConn3 -- SAG-MIC 247km/LConn3
  Cs CHMS/RConn3 -- CHM-JCA 2*252km/LConn3
  Cs CHMS/RConn2 -- CHM-JCA 2*252km/LConn2
  Cs CHMS/RConn1 -- CHM-JCA 2*252km/LConn1
  Cs SAG/RConn2 -- SAG-MIC 247km/LConn2
  SAG7/LConn2 -- CHM-SAG 117km/RConn2
  SAG7/LConn1 -- CHM-SAG 117km/RConn1
  SAG-MIC 247km/RConn1 -- North_East Network/LConn1
  SAG-MIC 247km/RConn2 -- North_East Network/LConn2
  SAG-MIC 247km/RConn3 -- North_East Network/LConn3
  QUE7/RConn1 -- North_East Network/LConn4
  QUE7/RConn2 -- North_East Network/LConn5
  QUE7/RConn3 -- North_East Network/LConn6
  MTL7/LConn1 -- MTL Load/LConn1 -- GFM_VC LCL_FILTER_VSC/RConn1 -- Load Flow Bus/LConn1 -- North-West Network/RConn1
  MTL7/LConn2 -- MTL Load/LConn2 -- GFM_VC LCL_FILTER_VSC/RConn2 -- North-West Network/RConn2
  MTL7/LConn3 -- MTL Load/LConn3 -- GFM_VC LCL_FILTER_VSC/RConn3 -- North-West Network/RConn3

== system GFM_29bus/Cs CHMS ==
  note: B
  Ca : powerlib/Elements/Series RLC Branch  LConnTagsString=__new0  RConnTagsString=__new0  BranchType=C  Resistance=1.0  Inductance=1.0  SetiL0=off  InitialCurrent=0  Capacitance=Cs  Setx0=off  InitialVoltage=0  Measurements=None
  Cb : powerlib/Elements/Series RLC Branch  LConnTagsString=__new0  RConnTagsString=__new0  BranchType=C  Resistance=1.0  Inductance=1.0  SetiL0=off  InitialCurrent=0  Capacitance=Cs  Setx0=off  InitialVoltage=0  Measurements=None
  Cc : powerlib/Elements/Series RLC Branch  LConnTagsString=__new0  RConnTagsString=__new0  BranchType=C  Resistance=1.0  Inductance=1.0  SetiL0=off  InitialCurrent=0  Capacitance=Cs  Setx0=off  InitialVoltage=0  Measurements=None
  A : PMIOPort  Side=Left
  B : PMIOPort  Port=2  Side=Left
  C : PMIOPort  Port=3  Side=Left
  "A " : PMIOPort  Port=4  Side=Right
  "B " : PMIOPort  Port=5  Side=Right
  "C " : PMIOPort  Port=6  Side=Right
  connections:
  Cc/RConn1 -- "C "/RConn1
  C/RConn1 -- Cc/LConn1
  Cb/RConn1 -- "B "/RConn1
  B/RConn1 -- Cb/LConn1
  Ca/RConn1 -- "A "/RConn1
  A/RConn1 -- Ca/LConn1

== system GFM_29bus/Cs SAG ==
  note: B
  Ca : powerlib/Elements/Series RLC Branch  LConnTagsString=__new0  RConnTagsString=__new0  BranchType=C  Resistance=1.0  Inductance=1.0  SetiL0=off  InitialCurrent=0  Capacitance=Cs  Setx0=off  InitialVoltage=0  Measurements=None
  Cb : powerlib/Elements/Series RLC Branch  LConnTagsString=__new0  RConnTagsString=__new0  BranchType=C  Resistance=1.0  Inductance=1.0  SetiL0=off  InitialCurrent=0  Capacitance=Cs  Setx0=off  InitialVoltage=0  Measurements=None
  Cc : powerlib/Elements/Series RLC Branch  LConnTagsString=__new0  RConnTagsString=__new0  BranchType=C  Resistance=1.0  Inductance=1.0  SetiL0=off  InitialCurrent=0  Capacitance=Cs  Setx0=off  InitialVoltage=0  Measurements=None
  A : PMIOPort  Side=Left
  B : PMIOPort  Port=2  Side=Left
  C : PMIOPort  Port=3  Side=Left
  "A " : PMIOPort  Port=4  Side=Right
  "B " : PMIOPort  Port=5  Side=Right
  "C " : PMIOPort  Port=6  Side=Right
  connections:
  A/RConn1 -- Ca/LConn1
  Ca/RConn1 -- "A "/RConn1
  B/RConn1 -- Cb/LConn1
  Cb/RConn1 -- "B "/RConn1
  C/RConn1 -- Cc/LConn1
  Cc/RConn1 -- "C "/RConn1

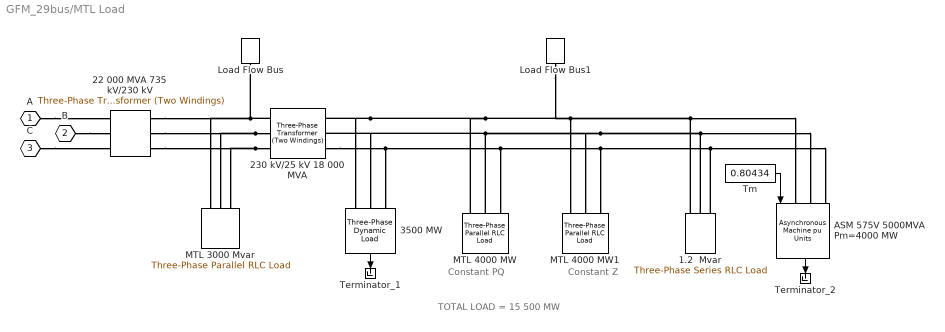
== system GFM_29bus/MTL Load ==
  note: Constant PQ
  note: Constant Z
  note: TOTAL LOAD = 15 500 MW
  1.2  Mvar : powerlib/Elements/Three-Phase Series RLC Load  LConnTagsString=A|B|C  Configuration=Y (grounded)  NominalVoltage=25e3  Vabc=[1e3 1e3 1e3]  Vabcp=[1e3 1e3 1e3]  NominalFrequency=60  UnbalancedPower=off  ActivePower=2000e6/50  InductivePower=0  CapacitivePower=2000e6  Pabc=[10e3 9e3 11e3]  QLabc=[100 90 110]  QCabc=[100 90 110]  Pabcp=[10e3 9e3 11e3]  QLabcp=[100 90 110]  QCabcp=[100 90 110]  Measurements=None  LoadType=constant Z
  22 000 MVA 735 kV/230 kV : powerlib/Elements/Three-Phase Transformer (Two Windings)  Winding1Connection=Yg  Winding2Connection=Delta (D1)  CoreType=Three single-phase transformers  SetSaturation=off  Hysteresis=off  DataFile='basic_model'  SetInitialFlux=off  Measurements=None  UNITS=pu  NominalPower=[ 22000e6 60 ]  Winding1="[ 735e3 0.002  0.12]"  Winding2=[230e3 0.002 0]  Rm=500  Lm=500  L0=0.5  Saturation="[ 0,0  ;  0.005,1.2  ;  1.0,1.4 ]"  InitialFluxes=[ 0.8 , -0.8 , 0.7 ]  BreakLoop=off  DiscreteSolver=Trapezoidal iterative  DataType=off  TransfoNumber=0
  230 kV/25 kV 18 000 MVA : powerlib/Elements/Three-Phase Transformer (Two Windings)  Winding1Connection=Yg  Winding2Connection=Delta (D1)  CoreType=Three single-phase transformers  SetSaturation=off  Hysteresis=off  DataFile='basic_model'  SetInitialFlux=off  Measurements=None  UNITS=pu  NominalPower=[18000e6 60 ]  Winding1="[ 230e3  0.08/30   0.08 ]"  Winding2="[ 25e3  0.08/30  0.08]"  Rm=500  Lm=500  L0=0.5  Saturation="[ 0,0  ;  0.005,1.2  ;  1.0,1.4 ]"  InitialFluxes=[ 0.8 , -0.8 , 0.7 ]  BreakLoop=off  DiscreteSolver=Trapezoidal iterative  DataType=off  TransfoNumber=0
  3500 MW : powerlib/Elements/Three-Phase Dynamic Load  NominalVoltage=[ 25e3 60 ]  ActiveReactivePowers=[3.5e+09 -7.63278e-08]  PositiveSequence=[0.977579 -90.0235]  ExternalControl=off  NpNq="[1.5  2.5]"  TimeConstants="[0  0  0  0]"  MinimumVoltage=0.7  Tfilter=1e-4  LoadFlowParameters=[4,0,0,0,0]
      settings: SourceProductBaseCode=PS
  ASM 575V 5000MVA Pm=4000 MW : powerlib/Machines/Asynchronous Machine pu Units  RotorType=Squirrel-cage  PresetModel=No  MechanicalLoad=Torque Tm  ShowDetailedParameters=on  ReferenceFrame=Rotor  Units=pu  MeasurementBus=off  NominalParameters="[5000e6 25e3  60]"  VoltageRatio=1  Stator=[0.01117 0.04832]  Rotor=[0.006 0.04832]  Cage1=[0.01909 0.0397]  Cage2=[0.01909 0.0397]  Lm=2.424  Mechanical="[1  0   2]"  PolePairs=2  InitialConditions=[0.00539423 0 0.951058 0.951058 0.951058 -118.861 -238.861 1.13934]  SimulateSaturation=off  Saturation="[0.212,0.4201,0.8125,1.0979,1.4799,2.2457,3.2586,4.5763,6.4763 ;   0.5,0.7,0.9,1,1.1,1.2 ,1.3,1.4,1.5]"  LoadFlowParameters=0  TsPowergui=0  TsBlock=-1  IterativeModel=Trapezoidal non iterative  IterativeDiscreteModel=Trapezoidal non iterative  Pmec=4000000000
      settings: SourceProductBaseCode=PS
  Load Flow Bus : powerlib/Measurements/Load Flow Bus  LConnTagsString=a  Phases=single  Connectors=on one side  ID=MTL2  Vbase=230e3  Vref=1  Vangle=0  VLF=0.9954  VLFb=1  VLFc=1  angleLF=-51.92  angleLFb=0  angleLFc=0
      settings: AttributesFormatString=%<ID>\n%<Vbase>V\n%<VLF>pu\n%<angleLF>deg.
  Load Flow Bus1 : powerlib/Measurements/Load Flow Bus  LConnTagsString=a  Phases=single  Connectors=on one side  ID=MTL_25  Vbase=25e3  Vref=1  Vangle=0  VLF=0.9776  VLFb=1  VLFc=1  angleLF=-90.02  angleLFb=0  angleLFc=0
      settings: AttributesFormatString=%<ID>\n%<Vbase>V\n%<VLF>pu\n%<angleLF>deg.
  MTL 3000 Mvar : powerlib/Elements/Three-Phase Parallel RLC Load  LConnTagsString=A|B|C  Configuration=Y (grounded)  NominalVoltage=230e3  Vabc=[1e3 1e3 1e3]  Vabcp=[1e3 1e3 1e3]  NominalFrequency=60  UnbalancedPower=off  ActivePower=0  InductivePower=0  CapacitivePower=3000e6  Pabc=[10e3 9e3 11e3]  QLabc=[100 90 110]  QCabc=[100 90 110]  Pabcp=[10e3 9e3 11e3]  QLabcp=[100 90 110]  QCabcp=[100 90 110]  Measurements=None  LoadType=constant Z
  MTL 4000 MW : powerlib/Elements/Three-Phase Parallel RLC Load  LConnTagsString=A|B|C  Configuration=Y (grounded)  NominalVoltage=(25000)*0.977579  Vabc=[1e3 1e3 1e3]  Vabcp=[1e3 1e3 1e3]  NominalFrequency=60  UnbalancedPower=off  ActivePower=4000000000  InductivePower=0  CapacitivePower=0  Pabc=[10e3 9e3 11e3]  QLabc=[100 90 110]  QCabc=[100 90 110]  Pabcp=[10e3 9e3 11e3]  QLabcp=[100 90 110]  QCabcp=[100 90 110]  Measurements=None  LoadType=constant PQ
  MTL 4000 MW1 : powerlib/Elements/Three-Phase Parallel RLC Load  LConnTagsString=A|B|C  Configuration=Y (grounded)  NominalVoltage=25e3  Vabc=[1e3 1e3 1e3]  Vabcp=[1e3 1e3 1e3]  NominalFrequency=60  UnbalancedPower=off  ActivePower=4000000000  InductivePower=0  CapacitivePower=0  Pabc=[10e3 9e3 11e3]  QLabc=[100 90 110]  QCabc=[100 90 110]  Pabcp=[10e3 9e3 11e3]  QLabcp=[100 90 110]  QCabcp=[100 90 110]  Measurements=None  LoadType=constant Z
  Terminator_1 : Terminator
  Terminator_2 : Terminator
  Tm : Constant  Value=0.80434
  A : PMIOPort  Side=Left
  B : PMIOPort  Port=2  Side=Left
  C : PMIOPort  Port=3  Side=Left
  wires:
  Tm/1 -> ASM 575V 5000MVA Pm=4000 MW/1
  3500 MW/1 -> Terminator_1/1
  ASM 575V 5000MVA Pm=4000 MW/1 -> Terminator_2/1
  connections:
  A/RConn1 -- 22 000 MVA 735 kV/230 kV/LConn1
  B/RConn1 -- 22 000 MVA 735 kV/230 kV/LConn2
  C/RConn1 -- 22 000 MVA 735 kV/230 kV/LConn3
  230 kV/25 kV 18 000 MVA/LConn1 -- Load Flow Bus/LConn1 -- 22 000 MVA 735 kV/230 kV/RConn1 -- MTL 3000 Mvar/LConn1
  230 kV/25 kV 18 000 MVA/LConn2 -- 22 000 MVA 735 kV/230 kV/RConn2 -- MTL 3000 Mvar/LConn2
  230 kV/25 kV 18 000 MVA/LConn3 -- 22 000 MVA 735 kV/230 kV/RConn3 -- MTL 3000 Mvar/LConn3
  MTL 4000 MW1/LConn1 -- Load Flow Bus1/LConn1 -- MTL 4000 MW/LConn1 -- 230 kV/25 kV 18 000 MVA/RConn1 -- 3500 MW/LConn1 -- ASM 575V 5000MVA Pm=4000 MW/LConn1 -- 1.2  Mvar/LConn1
  MTL 4000 MW1/LConn2 -- MTL 4000 MW/LConn2 -- 230 kV/25 kV 18 000 MVA/RConn2 -- 3500 MW/LConn2 -- ASM 575V 5000MVA Pm=4000 MW/LConn2 -- 1.2  Mvar/LConn2
  230 kV/25 kV 18 000 MVA/RConn3 -- ASM 575V 5000MVA Pm=4000 MW/LConn3 -- 1.2  Mvar/LConn3 -- MTL 4000 MW1/LConn3 -- MTL 4000 MW/LConn3 -- 3500 MW/LConn3

== system GFM_29bus/Model Initialization ==
